simulink model "c9mvofuz"  (R2022a)
settings: Solver=ode3  StartTime=0.0  StopTime=30.0  FixedStep=T  RelTol=1e-3  EnableMultiTasking=on
PreLoadFcn:
  | kp=1.1202;
  | ki=0.4391;
  | kd=2.0016;
  | lam=0.8647;
  | mu=1.0877;
  | T=0.001;
  | ffuz=readfis('voffuzzy');
  | fx0=[1 0.5 2.1 1 1]';
undefined symbols (not defined in the file): fuz, G, Gc, K0, N, ww
libraries: cstblocks x2
settings Model: Creator=liulu  LastModifiedBy=xuedi
settings SolverCC: AlgebraicLoopSolver=TrustRegion
settings DataIOCC: SaveFormat=Array  ReturnWorkspaceOutputs=off
settings OptimizationCC: LifeSpan=inf
settings DebuggingCC: UnderspecifiedInitializationDetection=Classic  MergeDetectMultiDrivingBlocksExec=none  SolverPrmCheckMsg=warning  FcnCallInpInsideContextMsg=warning  UnconnectedInputMsg=warning  UnconnectedOutputMsg=warning  UnconnectedLineMsg=warning  StateNameClashWarn=warning  SFUnexpectedBacktrackingDiag=warning  SFNoUnconditionalDefaultTransitionDiag=warning  SFExecutionAtInitializationDiag=none  SFMachineParentedDataDiag=warning  ArithmeticOperatorsInVariantConditions=warning
settings HardwareCC: ProdBitPerPointer=32  ProdBitPerSizeT=32  ProdBitPerPtrDiffT=32  ProdLargestAtomicFloat=None  ProdIntDivRoundTo=Undefined  ProdEndianess=Unspecified  ProdWordSize=32  ProdHWDeviceType=32-bit Generic
settings ModelReferenceCC: PropagateSignalLabelsOutOfModel=off
settings SFSimCC: SimUseLocalCustomCode=off  CustomCodeUndefinedFunction=UseInterfaceOnly
settings RTWCC: RTWUseLocalCustomCode=off
settings CodeAppCC: StateflowObjectComments=on
settings GRTTargetCC: TargetLangStandard=C89/C90 (ANSI)  CombineOutputUpdateFcns=off  GRTInterface=on
settings ConfigComp: CovMetricSettings=dw  CovSaveCumulativeToWorkspaceVar=on  CovSaveSingleToWorkspaceVar=on  CovExternalEMLEnable=off

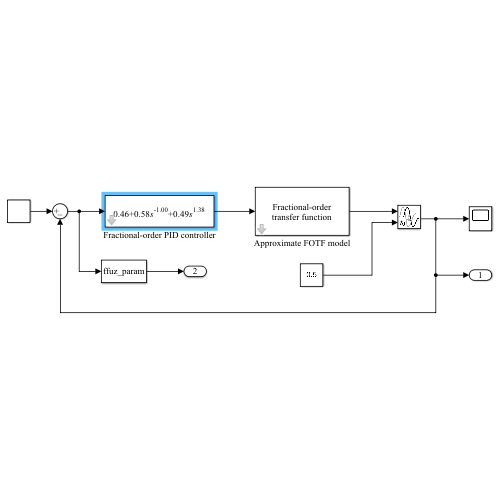
[thumbnail: Simulink's stored preview of the top-level diagram]
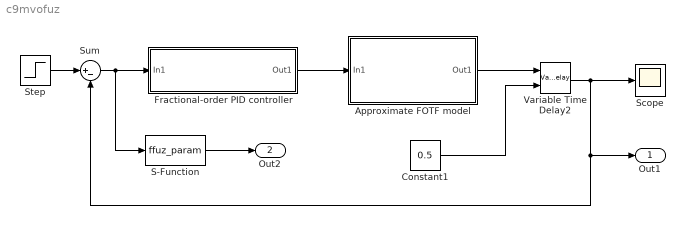
== system c9mvofuz ==
  Approximate FOTF model : Subsystem  mask{na=G, a=[1 3.3 2.9 3.32 1], nb=0, b=1, N=9, ww=[1e-5 1e3], kF=Oustaloup filter, T=0}
      mask prompts: na "Orders of the denominator"; a "Coefficients of the denominator"; nb "Orders of the numerator"; b "Coefficients of the numerator"; N "Filter order"; ww "Interested frequency range [wb wh]"; kF "Types of the filter"; T "Delay constant T"
      mask init:
      | if isa(na,'fotf'), G=na; T=G.ioDelay;
      | else
      |     if length(na)~=length(a), errordlg('Error','Mismatch on the denominator'), end
      |     if length(b)~=length(nb), errordlg('Error','Mismatch on the denominator'), end
      |     G=fotf(a,na,b,nb,T); 
      | end
      | if kF==1, str='ousta_fod'; else, str='new_fod'; end
      | wb=ww(1); wh=ww(2);
      | G1=high_order(G,str,wb,wh,N); G1.ioDelay=T;
      mask TypeOptions kF: Oustaloup filter | Modified Oustaloup filter
      mask Display: disp('Fractional-order\ntransfer function')
  Constant1 : Constant  Value=0.5
  Fractional-order PID controller : Subsystem  mask{Kp=Gc, II=[0.4391 0.8647], DD=[1.1907 0.3844], N=N, ww=ww, kFilter=Oustaloup filter}
      mask prompts: Kp "Proportional Kp"; II "Integral [Ki lam]"; DD "Differentiation [Kd mu]"; N "Filter order"; ww "Interested frequency range [wb wh]"; kFilter "Types of the filter"
      mask init:
      | if isa(Kp,'fotf'), a=Kp;
      |    lam=a.den.na; mu=a.num.na; mu=mu(1)-lam; b=a.num.a; Kd=b(1); Kp=b(2); Ki=b(3);
      | else, II=[II 1]; DD=[DD 1]; Ki=II(1); lam=II(2); Kd=DD(1); mu=DD(2); end
      | s=fotf('s'); a=Kp+Ki/s^lam+Kd*s^mu/(0.001*s+1);
      | Gc=high_order(a,'ousta_fod',ww(1),ww(2),N);
      | if abs(Ki)>0, sI=[sprintf('%.2f',Ki),'{\its}^{' sprintf('%.2f',-lam), '}']; end
      | if abs(Kd)>0, sD=[sprintf('%.2f',Kd),'{\its}^{' sprintf('%.2f',mu), '}']; end
      | str=sprintf('%.2f',Kp);
      | if abs(Ki)>0, if sI(1)~='-', sI=['+' sI]; end, str=[str,sI]; end
      | if abs(Kd)>0, if sD(1)~='-', sD=['+' sD]; end, str=[str,sD]; end
      mask TypeOptions kFilter: Oustaloup filter | Modified Oustaloup filter
      mask Display: disp(str,'texmode','on')
  S-Function : S-Function  FunctionName=ffuz_param  Parameters=T,fuz,K0  SFunctionDeploymentMode=off  EnableBusSupport=off
  Scope : Scope
  Step : Step  Time=0  SampleTime=0
  Sum : Sum  Inputs=|+-
  Variable Time Delay2 : VariableTransportDelay  MaximumDelay=10
  Out1 : Outport
  Out2 : Outport  Port=2
  wires:
  Step/1 -> Sum/1
  S-Function/1 -> Out2/1
  Constant1/1 -> Variable Time Delay2/2
  Approximate FOTF model/1(Out1) -> Variable Time Delay2/1
  Sum/1 -> Fractional-order PID controller/1(In1), S-Function/1
  Variable Time Delay2/1 -> Sum/2, Out1/1, Scope/1
  Fractional-order PID controller/1(Out1) -> Approximate FOTF model/1(In1)

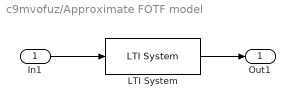
== system c9mvofuz/Approximate FOTF model ==
  In1 : Inport
  LTI System : cstblocks/LTI System  SystemSampleTime=-1  sys=G1  IC=[]
  Out1 : Outport
  wires:
  LTI System/1 -> Out1/1
  In1/1 -> LTI System/1

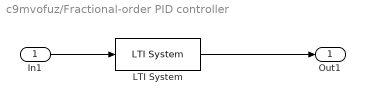
== system c9mvofuz/Fractional-order PID controller ==
  In1 : Inport
  LTI System : cstblocks/LTI System  sys=Gc  IC=[]
  Out1 : Outport
  wires:
  In1/1 -> LTI System/1
  LTI System/1 -> Out1/1
